simulink model "DIAGRAMA"  (R2021a)
settings: Solver=VariableStepAuto  StartTime=0.0  StopTime=10.0  RelTol=1e-3  EnableMultiTasking=on
settings Model: Creator=ACER  LastModifiedBy=ACER
settings SolverCC: AlgebraicLoopSolver=TrustRegion
settings DataIOCC: ReturnWorkspaceOutputs=off
settings OptimizationCC: LifeSpan=inf
settings DebuggingCC: SFUnexpectedBacktrackingDiag=warning  SFNoUnconditionalDefaultTransitionDiag=warning  SFMachineParentedDataDiag=warning  ArithmeticOperatorsInVariantConditions=warning
settings SFSimCC: SimUseLocalCustomCode=off  CustomCodeUndefinedFunction=UseInterfaceOnly
settings RTWCC: RTWUseLocalCustomCode=off
settings CodeAppCC: StateflowObjectComments=on
settings GRTTargetCC: TargetLangStandard=C89/C90 (ANSI)
settings ConfigComp: CovMetricSettings=dw  CovSaveCumulativeToWorkspaceVar=on  CovSaveSingleToWorkspaceVar=on  CovExternalEMLEnable=off

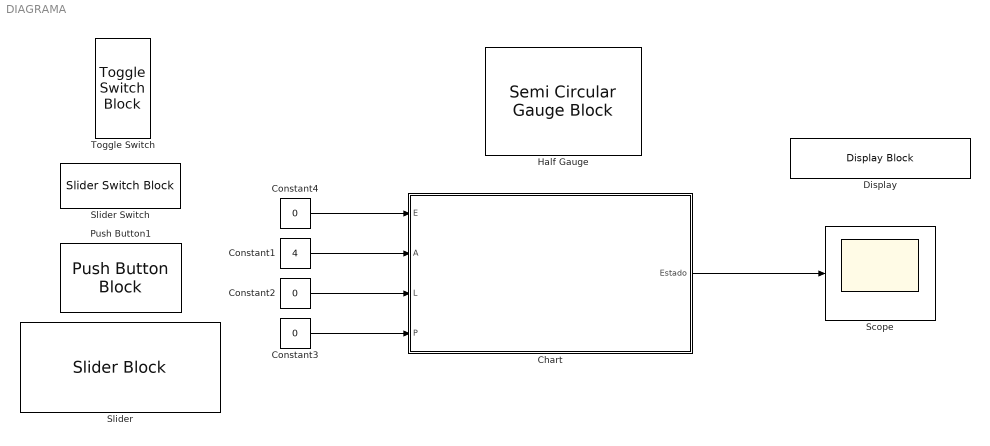
== system DIAGRAMA ==
  Chart : Stateflow chart  TreatAsAtomicUnit=on
  Constant1 : Constant  Value=4
  Constant2 : Constant  Value=0
  Constant3 : Constant  Value=0
  Constant4 : Constant  Value=0
  Display : DisplayBlock  LabelPosition=Hide  Format=short  Transparency=1
  Half Gauge : SemiCircularGaugeBlock
  Push Button1 : PushButtonBlock
  Scope : Scope
  Slider : SliderBlock  ScaleMax=4  TickInterval=1
  Slider Switch : SliderSwitchBlock
      settings: Values={{'Off', 'On'}, [0 1]}
  Toggle Switch : ToggleSwitchBlock
      settings: Values={{'Off', 'On'}, [0 1]}
  wires:
  Chart/1(Estado) -> Scope/1
  Constant1/1 -> Chart/2(A)
  Constant2/1 -> Chart/3(L)
  Constant3/1 -> Chart/4(P)
  Constant4/1 -> Chart/1(E)

== stateflow chart DIAGRAMA/Chart ==
  state S2
    entry: Estado = 2;
  state S1
    entry:
    Estado = 1;
  state S0
    entry:
    Estado = 0;
  state S4
    entry: Estado = 4;
  state S3
    entry: Estado = 3;
  S1 -> S2 [order 1] : [A == 1]
  S0 -> S1 : [E==1]
  S2 -> S1 : [A == 0]
  S1 -> S4 [order 3] : [L == 1]
  (default) -> S0
  S4 -> S1 : [L == 0]
  S1 -> S3 [order 2] : [P == 1]
  S3 -> S1 : [P == 0]
  data: Estado output; E input; A input; L input; P input
